simulink model "five_bar_discrete_model_v_1"  (R2018b)
settings: Solver=ode45  StartTime=0.0  StopTime=tmax-0.001  FixedStep=1e-4  MaxStep=1e-4  RelTol=1e-3
values from neighbouring files (symbols this model uses):
  dt = 10e-3    (= 0.01)    [model_parameters_v_1.m]    (also in test_dynamics.m = 0.2; test_kinematics.m = 0.1)
  dt_controller = 1e-3    (= 0.001)    [model_parameters_v_1.m]
  g = -9.80665    [idyn5.m]    (also in test_dynamics.m; test_model.m = 9.80665)
  Kd = (3*aj*wj-Fv) * eye(2)    [model_parameters_v_1.m]
  Kdi = [2 * zita *  wpos1; 2  * zita * wpos2]    [model_parameters_v_1.m]
  Ki = aj*wj^3 * eye(2)    [model_parameters_v_1.m]
  Kp = 3*aj*wj^2 * eye(2)    [model_parameters_v_1.m]
  Kpi = [ wpos1^2;  wpos2^2]    [model_parameters_v_1.m]
  lambda = 0.95    [model_parameters_v_1.m]
  p = [NaN; NaN]    [fkine5.m]    (also in test_model.m = zeros(n,2))
  q = [NaN; NaN; NaN; NaN; NaN]    [fkine5.m]    (also in ikine5.m = [q11;q12;q13;q21;q22])
  q0 = q(:,1)    [model_parameters_v_1.m]    (also in test_dynamics.m = q0(:,4); test_kinematics.m = q0(:,4))
  qd = [qda(1);qdu(1);qdu(2);qda(2);qdu(3)]    [ifirstkine5.m]
  qdd = [qdda(1);qddu(1);qddu(2);qdda(2);qddu(3)]    [isecondkine5.m]
  t0r = J * qda    [ffirstkine5.m]    (also in test_dynamics.m = [0;0]; test_kinematics.m = [1;1]; test_model.m = p)
  t0rd = (J * qdda+ at)    [fsecondkine5.m]    (also in test_dynamics.m = [0;0]; test_kinematics.m = [-1;1]; test_model.m = p)
undefined symbols (not defined in the file or in its folder): DiscIntNeverNeededParam, tmax, X, Y, Z
libraries: sm_lib x24, simulink x12, nesl_utility x9, commrandsrc3 x6, powerlib_meascontrol x2
(part 1 of 2)
settings Model: Creator=jere  LastModifiedBy=Jere
settings DebuggingCC: LibraryContextMissingDiagnostic=none
settings SFSimCC: SimUseLocalCustomCode=off
settings RTWCC: RTWUseLocalCustomCode=off

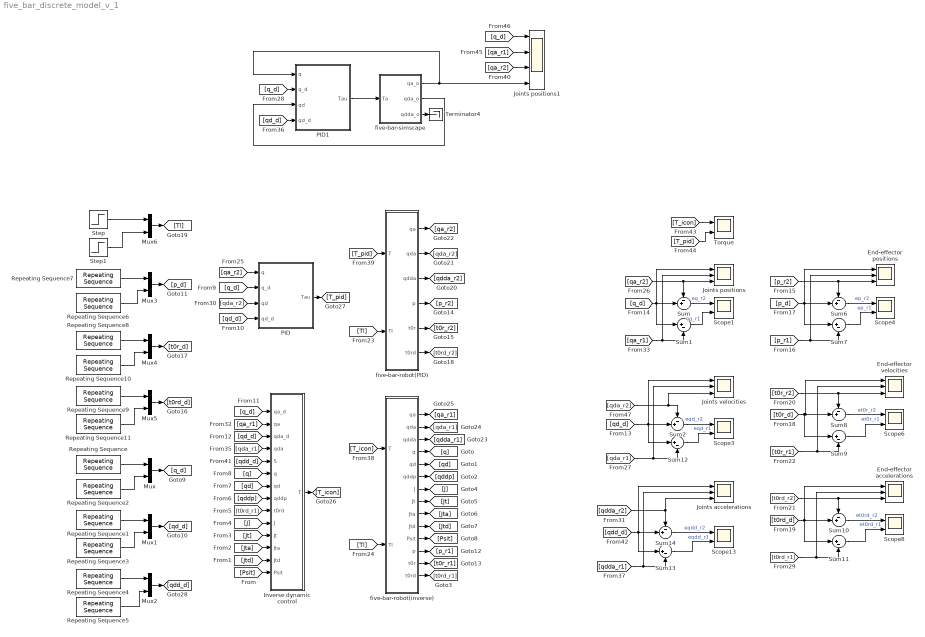
== system five_bar_discrete_model_v_1 ==
  End-effector accelerations : Scope  NumInputPorts=3
  End-effector positions : Scope  NumInputPorts=3
  End-effector velocities : Scope  NumInputPorts=3
  Inverse dynamic control : Subsystem
  Joints accelerations : Scope  NumInputPorts=3
  Joints positions : Scope  NumInputPorts=3
  Joints positions1 : Scope  NumInputPorts=4
  Joints velocities : Scope  NumInputPorts=3
  Mux{,1..6} (7 alike) : Mux  Inputs=2
  PID : Subsystem
  PID1 : Subsystem
  Repeating Sequence : simulink/Sources/Repeating Sequence  rep_seq_t=0:dt:tmax  rep_seq_y=q(1,:)
  Repeating Sequence1 : simulink/Sources/Repeating Sequence  rep_seq_t=0:dt:tmax  rep_seq_y=qd(1,:)
  Repeating Sequence10 : simulink/Sources/Repeating Sequence  rep_seq_t=0:dt:tmax  rep_seq_y=t0r(2,:)
  Repeating Sequence11 : simulink/Sources/Repeating Sequence  rep_seq_t=0:dt:tmax  rep_seq_y=t0rd(2,:)
  Repeating Sequence2 : simulink/Sources/Repeating Sequence  rep_seq_t=0:dt:tmax  rep_seq_y=q(4,:)
  Repeating Sequence3 : simulink/Sources/Repeating Sequence  rep_seq_t=0:dt:tmax  rep_seq_y=qd(4,:)
  Repeating Sequence4 : simulink/Sources/Repeating Sequence  rep_seq_t=0:dt:tmax  rep_seq_y=qdd(1,:)
  Repeating Sequence5 : simulink/Sources/Repeating Sequence  rep_seq_t=0:dt:tmax  rep_seq_y=qdd(4,:)
  Repeating Sequence6 : simulink/Sources/Repeating Sequence  rep_seq_t=0:dt:tmax  rep_seq_y=p(2,:)
  Repeating Sequence7 : simulink/Sources/Repeating Sequence  rep_seq_t=0:dt:tmax  rep_seq_y=p(1,:)
  Repeating Sequence8 : simulink/Sources/Repeating Sequence  rep_seq_t=0:dt:tmax  rep_seq_y=t0r(1,:)
  Repeating Sequence9 : simulink/Sources/Repeating Sequence  rep_seq_t=0:dt:tmax  rep_seq_y=t0rd(1,:)
  Scope{1,3..4,6,8,13} (6 alike) : Scope  NumInputPorts=2
  Step : Step  Time=tmax/2  SampleTime=0
  Step1 : Step  Time=tmax/2  SampleTime=0
  Sum{,2,6,8,10,14} (6 alike) : Sum  Inputs=-+|
  Sum{1,7,9,11..13} (6 alike) : Sum  Inputs=|+-
  Terminator4 : Terminator
  Torque : Scope  NumInputPorts=2
  five-bar-robot(PID) : Subsystem
  five-bar-robot(inverse) : Subsystem
  five-bar-simscape : Subsystem
  wires:
  Repeating Sequence/1 -> Mux/1
  Repeating Sequence2/1 -> Mux/2
  Repeating Sequence1/1 -> Mux1/1
  Repeating Sequence3/1 -> Mux1/2
  Repeating Sequence4/1 -> Mux2/1
  Repeating Sequence5/1 -> Mux2/2
  five-bar-robot(inverse)/4(q) -> [q]
  five-bar-robot(inverse)/5(qd) -> [qd]
  five-bar-robot(inverse)/6(qddp) -> [qddp]
  five-bar-robot(inverse)/14(t0rd) -> [t0rd_r1]
  five-bar-robot(inverse)/7(J) -> [J]
  five-bar-robot(inverse)/8(Jt) -> [Jt]
  five-bar-robot(inverse)/9(Jta) -> [Jta]
  five-bar-robot(inverse)/10(Jtd) -> [Jtd]
  five-bar-robot(inverse)/11(Psit) -> [Psit]
  [q] -> Inverse dynamic control/6(q)
  [qd] -> Inverse dynamic control/7(qd)
  [t0rd_r1] -> Inverse dynamic control/9(t0rd)
  [J] -> Inverse dynamic control/10(J)
  [Jt] -> Inverse dynamic control/11(Jt)
  [Jta] -> Inverse dynamic control/12(Jta)
  [Jtd] -> Inverse dynamic control/13(Jtd)
  [Psit] -> Inverse dynamic control/14(Psit)
  [qddp] -> Inverse dynamic control/8(qddp)
  five-bar-robot(PID)/1(qa) -> [qa_r2]
  Sum/1 -> Scope1/1  "eq_r2"
  Sum1/1 -> Scope1/2  "eq_r1"
  Mux/1 -> [q_d]
  [q_d] -> PID/2(q_d)
  Mux1/1 -> [qd_d]
  [qd_d] -> PID/4(qd_d)
  [qd_d] -> Inverse dynamic control/3(qda_d)
  [q_d] -> Inverse dynamic control/1(qa_d)
  Repeating Sequence6/1 -> Mux3/2
  Repeating Sequence7/1 -> Mux3/1
  Mux3/1 -> [p_d]
  five-bar-robot(inverse)/12(p) -> [p_r1]
  five-bar-robot(inverse)/13(t0r) -> [t0r_r1]
  five-bar-robot(PID)/4(p) -> [p_r2]
  five-bar-robot(PID)/5(t0r) -> [t0r_r2]
  Sum6/1 -> Scope4/1  "ep_r2"
  Sum7/1 -> Scope4/2  "ep_r1"
  [p_d] -> End-effector positions/1, Sum6/2, Sum7/1
  [p_r2] -> End-effector positions/3, Sum6/1
  [p_r1] -> End-effector positions/2, Sum7/2
  Repeating Sequence11/1 -> Mux5/2
  Repeating Sequence9/1 -> Mux5/1
  Repeating Sequence8/1 -> Mux4/1
  Mux5/1 -> [t0rd_d]
  Mux4/1 -> [t0r_d]
  Repeating Sequence10/1 -> Mux4/2
  five-bar-robot(PID)/6(t0rd) -> [t0rd_r2]
  [t0r_r1] -> End-effector velocities/2, Sum9/2
  Sum9/1 -> Scope6/2  "et0r_r1"
  [t0r_d] -> Sum9/1, End-effector velocities/1, Sum8/2
  [t0r_r2] -> End-effector velocities/3, Sum8/1
  Sum8/1 -> Scope6/1  "et0r_r2"
  [t0rd_r1] -> End-effector accelerations/2, Sum11/2
  Sum11/1 -> Scope8/2  "et0rd_r1"
  [t0rd_d] -> End-effector accelerations/1, Sum10/2, Sum11/1
  [t0rd_r2] -> End-effector accelerations/3, Sum10/1
  Sum10/1 -> Scope8/1  "et0rd_r2"
  five-bar-robot(PID)/3(qdda) -> [qdda_r2]
  [Tl] -> five-bar-robot(PID)/2(Tl)
  [Tl] -> five-bar-robot(inverse)/2(Tl)
  Step/1 -> Mux6/1
  Step1/1 -> Mux6/2
  Mux6/1 -> [Tl]
  [qa_r2] -> PID/1(q)
  [qa_r2] -> Sum/1, Joints positions/3
  five-bar-robot(PID)/2(qda) -> [qda_r2]
  [q_d] -> Sum/2, Sum1/1, Joints positions/1
  [qda_r2] -> PID/3(qd)
  five-bar-robot(inverse)/1(qa) -> [qa_r1]
  [qa_r1] -> Inverse dynamic control/2(qa)
  [qa_r1] -> Sum1/2, Joints positions/2
  [qda_r1] -> Joints velocities/2, Sum12/2
  five-bar-robot(inverse)/2(qda) -> [qda_r1]
  [qda_r1] -> Inverse dynamic control/4(qda)
  five-bar-robot(inverse)/3(qdda) -> [qdda_r1]
  Inverse dynamic control/1(T) -> [T_icon]
  [T_icon] -> five-bar-robot(inverse)/1(T)
  PID/1(Tau) -> [T_pid]
  [T_pid] -> five-bar-robot(PID)/1(T)
  Mux2/1 -> [qdd_d]
  [qdd_d] -> Inverse dynamic control/5(qdda_d)
  [T_icon] -> Torque/1
  [T_pid] -> Torque/2
  Sum2/1 -> Scope3/1  "eqd_r2"
  Sum12/1 -> Scope3/2  "eqd_r1"
  [qd_d] -> Sum2/2, Sum12/1, Joints velocities/1
  [qda_r2] -> Joints velocities/3, Sum2/1
  Sum13/1 -> Scope13/2  "eqdd_r1"
  [qdd_d] -> Sum13/1, Joints accelerations/1, Sum14/2
  [qdda_r1] -> Sum13/2, Joints accelerations/2
  Sum14/1 -> Scope13/1  "eqdd_r2"
  [qdda_r2] -> Sum14/1, Joints accelerations/3
  PID1/1(Tau) -> five-bar-simscape/1(Ta)
  five-bar-simscape/1(qa_o) -> Joints positions1/4, PID1/1(q)
  five-bar-simscape/2(qda_o) -> PID1/3(qd)
  [q_d] -> PID1/2(q_d)
  [qd_d] -> PID1/4(qd_d)
  [q_d] -> Joints positions1/1
  [qa_r1] -> Joints positions1/2
  [qa_r2] -> Joints positions1/3
  five-bar-simscape/3(qdda_o) -> Terminator4/1

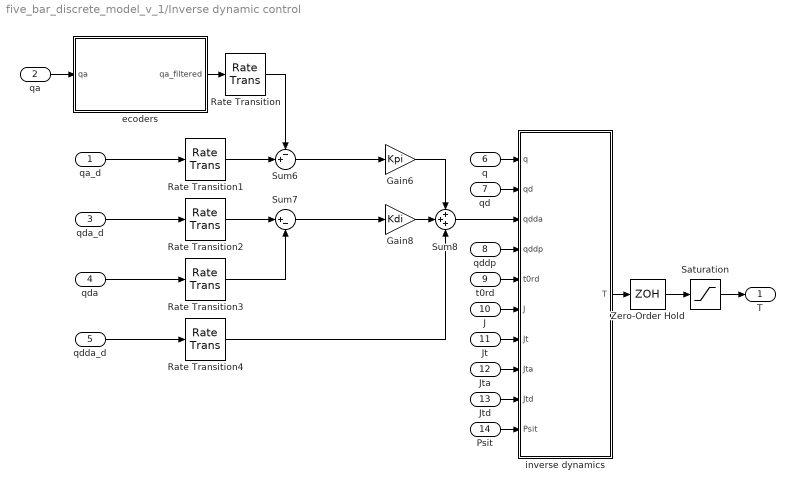
== system five_bar_discrete_model_v_1/Inverse dynamic control ==
  qa_d : Inport
  qa : Inport  Port=2
  qda_d : Inport  Port=3
  qda : Inport  Port=4
  qdda_d : Inport  Port=5
  q : Inport  Port=6
  qd : Inport  Port=7
  qddp : Inport  Port=8
  t0rd : Inport  Port=9
  J : Inport  Port=10
  Jt : Inport  Port=11
  Jta : Inport  Port=12
  Jtd : Inport  Port=13
  Psit : Inport  Port=14
  Gain6 : Gain  Gain=Kpi
  Gain8 : Gain  Gain=Kdi
  Rate Transition{,1..4} (5 alike) : RateTransition  InitialCondition=[q0(1);q0(4)]  OutPortSampleTime=dt_controller
  Saturation : Saturate  UpperLimit=3  LowerLimit=-3
  Sum6 : Sum  Inputs=-+|
  Sum7 : Sum  Inputs=|+-
  Sum8 : Sum  Inputs=+++
  Zero-Order Hold : ZeroOrderHold  SampleTime=dt_controller
  ecoders : Subsystem
  inverse dynamics : MATLAB Function  TreatAsAtomicUnit=on
  T : Outport
  wires:
  Psit/1 -> inverse dynamics/10(Psit)
  J/1 -> inverse dynamics/6(J)
  Sum7/1 -> Gain8/1
  Sum6/1 -> Gain6/1
  qa_d/1 -> Rate Transition1/1
  Jta/1 -> inverse dynamics/8(Jta)
  qd/1 -> inverse dynamics/2(qd)
  qddp/1 -> inverse dynamics/4(qddp)
  q/1 -> inverse dynamics/1(q)
  t0rd/1 -> inverse dynamics/5(t0rd)
  qdda_d/1 -> Rate Transition4/1
  inverse dynamics/1(T) -> Zero-Order Hold/1
  Jtd/1 -> inverse dynamics/9(Jtd)
  Jt/1 -> inverse dynamics/7(Jt)
  qda/1 -> Rate Transition3/1
  qda_d/1 -> Rate Transition2/1
  Gain8/1 -> Sum8/2
  Gain6/1 -> Sum8/1
  Saturation/1 -> T/1
  Sum8/1 -> inverse dynamics/3(qdda)
  Rate Transition/1 -> Sum6/1
  Rate Transition1/1 -> Sum6/2
  Rate Transition2/1 -> Sum7/1
  Rate Transition3/1 -> Sum7/2
  Rate Transition4/1 -> Sum8/3
  qa/1 -> ecoders/1(qa)
  ecoders/1(qa_filtered) -> Rate Transition/1
  Zero-Order Hold/1 -> Saturation/1

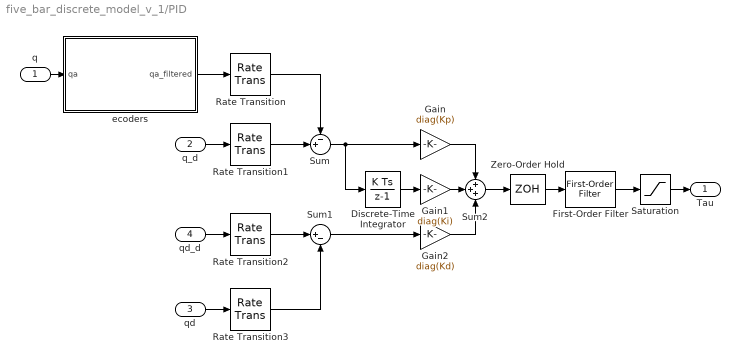
== system five_bar_discrete_model_v_1/PID ==
  q : Inport
  q_d : Inport  Port=2
  qd : Inport  Port=3
  qd_d : Inport  Port=4
  Discrete-Time Integrator : DiscreteIntegrator  InitialCondition=[0;0]  SampleTime=dt_controller  ICPrevOutput=DiscIntNeverNeededParam  ICPrevScaledInput=DiscIntNeverNeededParam
  First-Order Filter : powerlib_meascontrol/Filters/First-Order Filter  FilterType=Lowpass  Tc=0.006  Ts=dt_controller  Initialize=off  Vac_Init=[0, 0, 60]  Vdc_Init=0  PlotResponse=off  FreqRange="[0,  200,  1]"
      settings: SourceProductName=Simscape Electrical
  Gain : Gain  Gain=diag(Kp)
  Gain1 : Gain  Gain=diag(Ki)
  Gain2 : Gain  Gain=diag(Kd)
  Rate Transition{,1..3} (4 alike) : RateTransition  InitialCondition=[q0(1);q0(4)]  OutPortSampleTime=dt_controller
  Saturation : Saturate  UpperLimit=2  LowerLimit=-2
  Sum : Sum  Inputs=-+|
  Sum1 : Sum  Inputs=|+-
  Sum2 : Sum  Inputs=+++
  Zero-Order Hold : ZeroOrderHold  SampleTime=dt_controller
  ecoders : Subsystem
  Tau : Outport
  wires:
  Gain/1 -> Sum2/1
  Sum/1 -> Discrete-Time Integrator/1, Gain/1
  Gain1/1 -> Sum2/2
  q_d/1 -> Rate Transition1/1
  qd_d/1 -> Rate Transition2/1
  Sum2/1 -> Zero-Order Hold/1
  Sum1/1 -> Gain2/1
  qd/1 -> Rate Transition3/1
  Gain2/1 -> Sum2/3
  First-Order Filter/1 -> Saturation/1
  Saturation/1 -> Tau/1
  Rate Transition1/1 -> Sum/2
  Rate Transition2/1 -> Sum1/1
  Rate Transition3/1 -> Sum1/2
  Zero-Order Hold/1 -> First-Order Filter/1
  Discrete-Time Integrator/1 -> Gain1/1
  Rate Transition/1 -> Sum/1
  q/1 -> ecoders/1(qa)
  ecoders/1(qa_filtered) -> Rate Transition/1

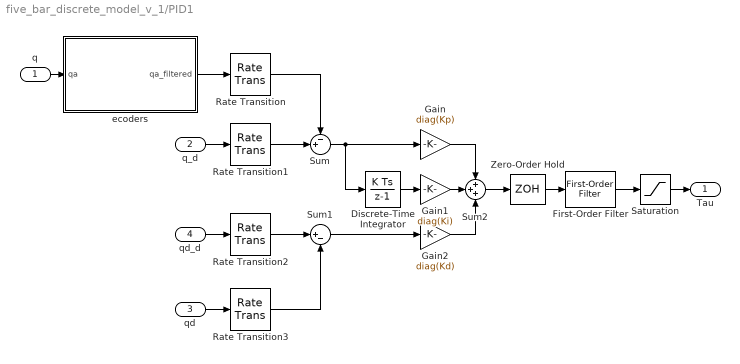
== system five_bar_discrete_model_v_1/PID1 ==
  q : Inport
  q_d : Inport  Port=2
  qd : Inport  Port=3
  qd_d : Inport  Port=4
  Discrete-Time Integrator : DiscreteIntegrator  InitialCondition=[0;0]  SampleTime=dt_controller  ICPrevOutput=DiscIntNeverNeededParam  ICPrevScaledInput=DiscIntNeverNeededParam
  First-Order Filter : powerlib_meascontrol/Filters/First-Order Filter  FilterType=Lowpass  Tc=0.006  Ts=dt_controller  Initialize=off  Vac_Init=[0, 0, 60]  Vdc_Init=0  PlotResponse=off  FreqRange="[0,  200,  1]"
      settings: SourceProductName=Simscape Electrical
  Gain : Gain  Gain=diag(Kp)
  Gain1 : Gain  Gain=diag(Ki)
  Gain2 : Gain  Gain=diag(Kd)
  Rate Transition{,1..3} (4 alike) : RateTransition  InitialCondition=[q0(1);q0(4)]  OutPortSampleTime=dt_controller
  Saturation : Saturate  UpperLimit=2  LowerLimit=-2
  Sum : Sum  Inputs=-+|
  Sum1 : Sum  Inputs=|+-
  Sum2 : Sum  Inputs=+++
  Zero-Order Hold : ZeroOrderHold  SampleTime=dt_controller
  ecoders : Subsystem
  Tau : Outport
  wires:
  Gain/1 -> Sum2/1
  Sum/1 -> Discrete-Time Integrator/1, Gain/1
  Gain1/1 -> Sum2/2
  q_d/1 -> Rate Transition1/1
  qd_d/1 -> Rate Transition2/1
  Sum2/1 -> Zero-Order Hold/1
  Sum1/1 -> Gain2/1
  qd/1 -> Rate Transition3/1
  Gain2/1 -> Sum2/3
  First-Order Filter/1 -> Saturation/1
  Saturation/1 -> Tau/1
  Rate Transition1/1 -> Sum/2
  Rate Transition2/1 -> Sum1/1
  Rate Transition3/1 -> Sum1/2
  Zero-Order Hold/1 -> First-Order Filter/1
  Discrete-Time Integrator/1 -> Gain1/1
  Rate Transition/1 -> Sum/1
  q/1 -> ecoders/1(qa)
  ecoders/1(qa_filtered) -> Rate Transition/1

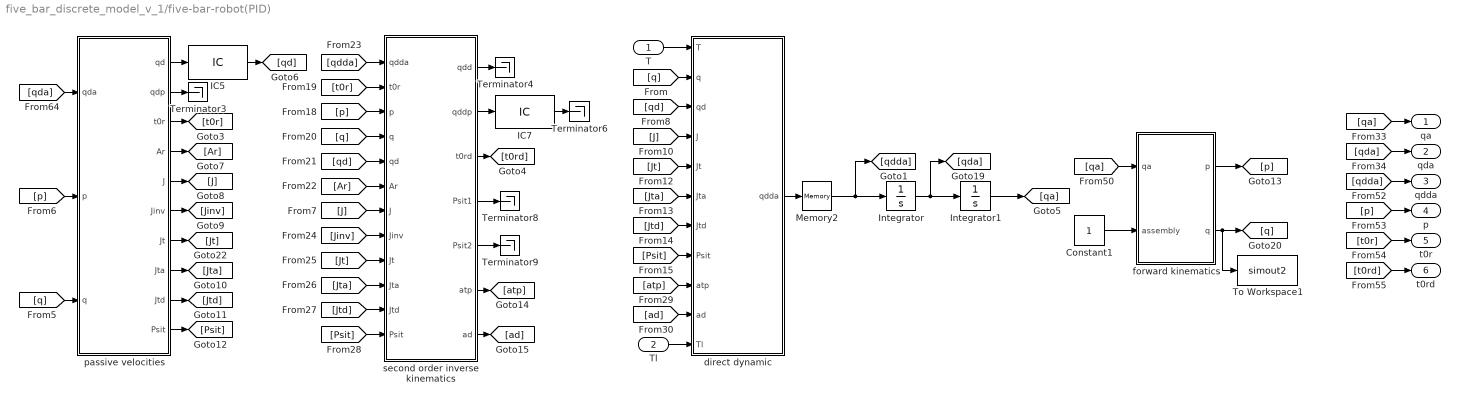
== system five_bar_discrete_model_v_1/five-bar-robot(PID) ==
  T : Inport
  Tl : Inport  Port=2
  Constant1 : Constant
  IC5 : InitialCondition  Value=zeros(5,1)
  IC7 : InitialCondition  Value=zeros(3,1)
  Integrator : Integrator  InitialCondition=[0;0]
  Integrator1 : Integrator  InitialCondition=[q0(1);q0(4)]
  Memory2 : Memory  InitialCondition=[0;0]
  Terminator{3..4,6,8..9} (5 alike) : Terminator
  To Workspace1 : ToWorkspace  VariableName=simout2  SaveFormat=Timeseries  SampleTime=-1
  direct dynamic : MATLAB Function  TreatAsAtomicUnit=on
  forward kinematics : MATLAB Function  TreatAsAtomicUnit=on
  passive velocities : MATLAB Function  TreatAsAtomicUnit=on
  second order inverse kinematics : MATLAB Function  TreatAsAtomicUnit=on
  qa : Outport
  qda : Outport  Port=2
  qdda : Outport  Port=3
  p : Outport  Port=4
  t0r : Outport  Port=5
  t0rd : Outport  Port=6
  wires:
  [qdda] -> qdda/1
  [qa] -> forward kinematics/1(qa)
  forward kinematics/1(p) -> [p]
  forward kinematics/2(q) -> To Workspace1/1, [q]
  Constant1/1 -> forward kinematics/2(assembly)
  [qda] -> qda/1
  [p] -> p/1
  [t0r] -> t0r/1
  [t0rd] -> t0rd/1
  [Jt] -> second order inverse kinematics/9(Jt)
  [Jtd] -> second order inverse kinematics/11(Jtd)
  [p] -> passive velocities/2(p)
  [qd] -> second order inverse kinematics/5(qd)
  Integrator1/1 -> [qa]
  second order inverse kinematics/5(Psit2) -> Terminator9/1
  passive velocities/3(t0r) -> [t0r]
  [Jta] -> second order inverse kinematics/10(Jta)
  [atp] -> direct dynamic/9(atp)
  T/1 -> direct dynamic/1(T)
  second order inverse kinematics/7(ad) -> [ad]
  passive velocities/1(qd) -> IC5/1
  second order inverse kinematics/4(Psit1) -> Terminator8/1
  Integrator/1 -> [qda], Integrator1/1
  passive velocities/6(Jinv) -> [Jinv]
  [J] -> second order inverse kinematics/7(J)
  passive velocities/8(Jta) -> [Jta]
  [Ar] -> second order inverse kinematics/6(Ar)
  second order inverse kinematics/6(atp) -> [atp]
  passive velocities/4(Ar) -> [Ar]
  [Jta] -> direct dynamic/6(Jta)
  [qdda] -> second order inverse kinematics/1(qdda)
  [qda] -> passive velocities/1(qda)
  [q] -> second order inverse kinematics/4(q)
  [p] -> second order inverse kinematics/3(p)
  Memory2/1 -> Integrator/1, [qdda]
  IC7/1 -> Terminator6/1
  [t0r] -> second order inverse kinematics/2(t0r)
  [q] -> direct dynamic/2(q)
  second order inverse kinematics/3(t0rd) -> [t0rd]
  passive velocities/7(Jt) -> [Jt]
  [q] -> passive velocities/3(q)
  [Jt] -> direct dynamic/5(Jt)
  Tl/1 -> direct dynamic/11(Tl)
  [ad] -> direct dynamic/10(ad)
  [qd] -> direct dynamic/3(qd)
  passive velocities/10(Psit) -> [Psit]
  [Jtd] -> direct dynamic/7(Jtd)
  passive velocities/2(qdp) -> Terminator3/1
  [Psit] -> second order inverse kinematics/12(Psit)
  direct dynamic/1(qdda) -> Memory2/1
  second order inverse kinematics/2(qddp) -> IC7/1
  [Jinv] -> second order inverse kinematics/8(Jinv)
  [Psit] -> direct dynamic/8(Psit)
  IC5/1 -> [qd]
  [J] -> direct dynamic/4(J)
  second order inverse kinematics/1(qdd) -> Terminator4/1
  passive velocities/5(J) -> [J]
  passive velocities/9(Jtd) -> [Jtd]
  [qa] -> qa/1

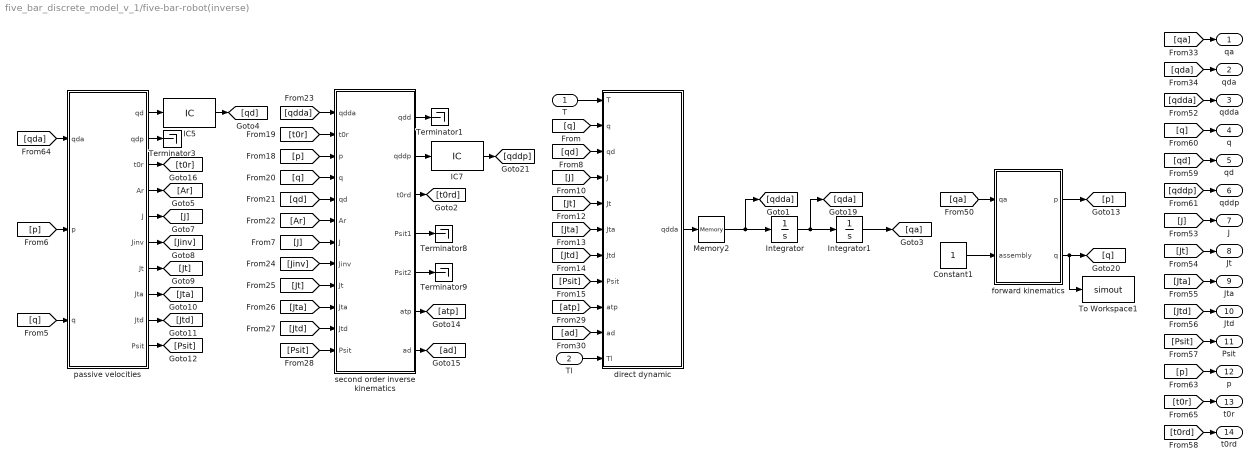
== system five_bar_discrete_model_v_1/five-bar-robot(inverse) ==
  T : Inport
  Tl : Inport  Port=2
  Constant1 : Constant
  IC5 : InitialCondition  Value=zeros(5,1)
  IC7 : InitialCondition  Value=zeros(3,1)
  Integrator : Integrator  InitialCondition=[0;0]
  Integrator1 : Integrator  InitialCondition=[q0(1);q0(4)]
  Memory2 : Memory  InitialCondition=[0;0]
  Terminator{1,3,8..9} (4 alike) : Terminator
  To Workspace1 : ToWorkspace  VariableName=simout  SaveFormat=Timeseries  SampleTime=-1
  direct dynamic : MATLAB Function  TreatAsAtomicUnit=on
  forward kinematics : MATLAB Function  TreatAsAtomicUnit=on
  passive velocities : MATLAB Function  TreatAsAtomicUnit=on
  second order inverse kinematics : MATLAB Function  TreatAsAtomicUnit=on
  qa : Outport
  qda : Outport  Port=2
  qdda : Outport  Port=3
  q : Outport  Port=4
  qd : Outport  Port=5
  qddp : Outport  Port=6
  J : Outport  Port=7
  Jt : Outport  Port=8
  Jta : Outport  Port=9
  Jtd : Outport  Port=10
  Psit : Outport  Port=11
  p : Outport  Port=12
  t0r : Outport  Port=13
  t0rd : Outport  Port=14
  wires:
  [p] -> second order inverse kinematics/3(p)
  second order inverse kinematics/6(atp) -> [atp]
  [ad] -> direct dynamic/10(ad)
  [Psit] -> second order inverse kinematics/12(Psit)
  [q] -> second order inverse kinematics/4(q)
  passive velocities/7(Jt) -> [Jt]
  [qd] -> direct dynamic/3(qd)
  [Psit] -> direct dynamic/8(Psit)
  [Jinv] -> second order inverse kinematics/8(Jinv)
  passive velocities/10(Psit) -> [Psit]
  Integrator1/1 -> [qa]
  passive velocities/4(Ar) -> [Ar]
  second order inverse kinematics/5(Psit2) -> Terminator9/1
  second order inverse kinematics/7(ad) -> [ad]
  [qdda] -> qdda/1
  [qd] -> second order inverse kinematics/5(qd)
  [Jta] -> direct dynamic/6(Jta)
  [q] -> direct dynamic/2(q)
  passive velocities/5(J) -> [J]
  passive velocities/6(Jinv) -> [Jinv]
  [qa] -> forward kinematics/1(qa)
  second order inverse kinematics/4(Psit1) -> Terminator8/1
  forward kinematics/1(p) -> [p]
  forward kinematics/2(q) -> To Workspace1/1, [q]
  passive velocities/9(Jtd) -> [Jtd]
  [Jta] -> second order inverse kinematics/10(Jta)
  [Jt] -> second order inverse kinematics/9(Jt)
  [t0r] -> second order inverse kinematics/2(t0r)
  Constant1/1 -> forward kinematics/2(assembly)
  [J] -> direct dynamic/4(J)
  [qa] -> qa/1
  [Jt] -> direct dynamic/5(Jt)
  [Ar] -> second order inverse kinematics/6(Ar)
  [Jtd] -> direct dynamic/7(Jtd)
  Integrator/1 -> [qda], Integrator1/1
  passive velocities/1(qd) -> IC5/1
  [q] -> passive velocities/3(q)
  passive velocities/8(Jta) -> [Jta]
  [p] -> passive velocities/2(p)
  [qda] -> qda/1
  passive velocities/2(qdp) -> Terminator3/1
  IC5/1 -> [qd]
  [Jtd] -> second order inverse kinematics/11(Jtd)
  T/1 -> direct dynamic/1(T)
  [atp] -> direct dynamic/9(atp)
  [q] -> q/1
  [qd] -> qd/1
  [qddp] -> qddp/1
  [t0rd] -> t0rd/1
  [J] -> J/1
  [Jt] -> Jt/1
  [Jta] -> Jta/1
  [Jtd] -> Jtd/1
  [Psit] -> Psit/1
  direct dynamic/1(qdda) -> Memory2/1
  [p] -> p/1
  [t0r] -> t0r/1
  Tl/1 -> direct dynamic/11(Tl)
  [qda] -> passive velocities/1(qda)
  [qdda] -> second order inverse kinematics/1(qdda)
  passive velocities/3(t0r) -> [t0r]
  [J] -> second order inverse kinematics/7(J)
  second order inverse kinematics/3(t0rd) -> [t0rd]
  second order inverse kinematics/2(qddp) -> IC7/1
  IC7/1 -> [qddp]
  Memory2/1 -> Integrator/1, [qdda]
  second order inverse kinematics/1(qdd) -> Terminator1/1

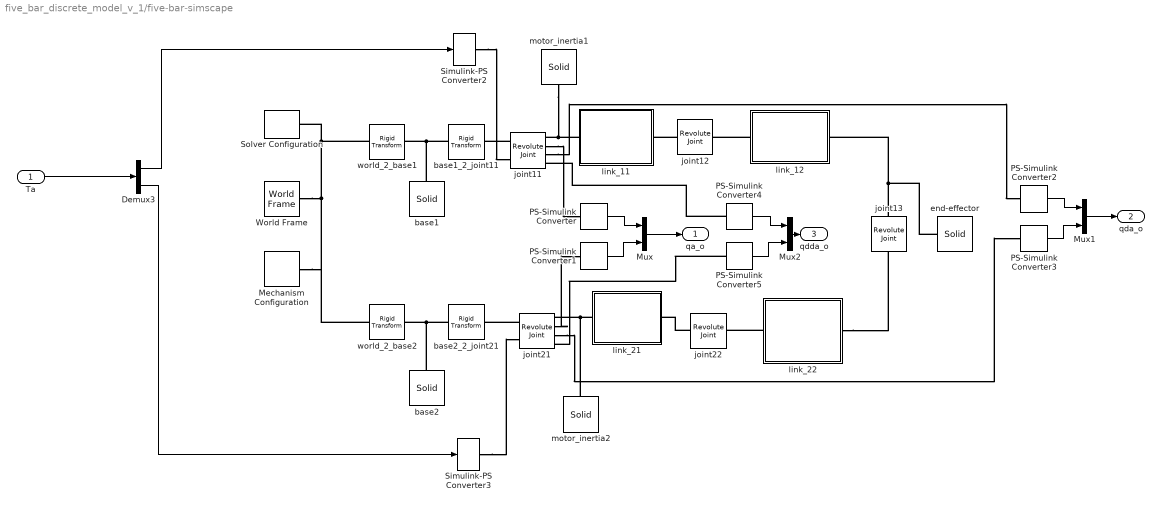
== system five_bar_discrete_model_v_1/five-bar-simscape ==
  Ta : Inport
  Demux3 : Demux  Outputs=2
  Mechanism Configuration : sm_lib/Utilities/Mechanism Configuration  UniformGravity=Constant  GravityVector=[0 0 0]  GravityUnits=m/s^2  LinearizationDelta=0.001
  Mux : Mux  Inputs=2
  Mux1 : Mux  Inputs=2
  Mux2 : Mux  Inputs=2
  PS-Simulink Converter : nesl_utility/PS-Simulink Converter  PhysicalDomain=network_engine_domain  SubClassName=ps_output  LeftPortType=input  RightPortType=output  PseudoPeriodic=off  Frequencies=[]  Unit=rad  AffineConversion=off
  PS-Simulink Converter1 : nesl_utility/PS-Simulink Converter  PhysicalDomain=network_engine_domain  SubClassName=ps_output  LeftPortType=input  RightPortType=output  PseudoPeriodic=off  Frequencies=[]  Unit=rad  AffineConversion=off
  PS-Simulink Converter{2..5} (4 alike) : nesl_utility/PS-Simulink Converter  PhysicalDomain=network_engine_domain  SubClassName=ps_output  LeftPortType=input  RightPortType=output  PseudoPeriodic=off  Frequencies=[]  Unit=1  AffineConversion=off
  Simulink-PS Converter2 : nesl_utility/Simulink-PS Converter  PhysicalDomain=network_engine_domain  SubClassName=ps_input  LeftPortType=input  RightPortType=output  PseudoPeriodic=off  Frequencies=[]  NoiseDistribution=none  NoiseParameters=[]  Unit=N*m  AffineConversion=off  FilteringAndDerivatives=provide  SimscapeFilterOrder=1  InputFilterTimeConstant=0.001  UdotUserProvided=0
  Simulink-PS Converter3 : nesl_utility/Simulink-PS Converter  PhysicalDomain=network_engine_domain  SubClassName=ps_input  LeftPortType=input  RightPortType=output  PseudoPeriodic=off  Frequencies=[]  NoiseDistribution=none  NoiseParameters=[]  Unit=N*m  AffineConversion=off  FilteringAndDerivatives=provide  SimscapeFilterOrder=1  InputFilterTimeConstant=0.001  UdotUserProvided=0
  Solver Configuration : nesl_utility/Solver Configuration  PhysicalDomain=network_engine_domain  SubClassName=solver  LeftPortType=input  RightPortType=generic  Tones=[]  Harmonics=[]  SimulateNoise=off  Profile=off  UseLocalSampling=off  EnableSwitchedLinearOptims=on  FrequencyDomain=off  UseCCode=off  RelTol=0.001  AbsTol=1e-06  MinStep=1e-09  ToWorkspace=off  RevertToSquareIcSolve=off  NumHomotopyIterations=100  PhasorMode=off  PhasorModeNumHarmonics=1  DoDC=off  ResidualTolerance=1e-09  UseLocalSolver=off  LocalSolverChoice=NE_BACKWARD_EULER_ADVANCER  LocalSolverSampleTime=0.001  DoFixedCost=off  MaxNonlinIter=3  MaxModeIter=2  LinearAlgebra=Sparse  EquationFormulation=NE_TIME_EF  DelaysMemoryBudget=1024  AutomaticFiltering=on  FilteringTimeConstant=0.001  PartitionStorageMethod=AS_NEEDED  PartitionMemoryBudget=1024
  World Frame : sm_lib/Frames and Transforms/World Frame
  base1 : sm_lib/Body Elements/Solid  InertiaType=PointMass  Mass=1.72  MassUnits=kg  CenterOfMass=[0 0 0]  CenterOfMassUnits=m  MomentsOfInertia=[1 1 1]  MomentsOfInertiaUnits=kg*m^2  ProductsOfInertia=[0 0 0]  ProductsOfInertiaUnits=kg*m^2  BasedOnType=Density  Density=1000  DensityUnits=kg/m^3  DoExposeReferenceFrame=on  SerializedFrames=<Frames/>  GraphicType=FromGeometry  MarkerShape=Sphere  MarkerSize=10  GraphicVisPropType=SimpleVisualProperties  GraphicDiffuseColor=[1.0 1.0 0.0]  GraphicSpecularColor=[0.5 0.5 0.5 1.0]  GraphicAmbientColor=[0.15 0.15 0.15 1.0]  GraphicEmissiveColor=[0.0 0.0 0.0 1.0]  GraphicShininess=75  GraphicOpacity=1.0  GeometryShape=FromFile  RectangleSize=[1 1]  RectangleSizeUnits=m  BrickDimensions=[1 1 1]  BrickDimensionUnits=m  CylinderRadius=1  CylinderRadiusUnits=m  CylinderLength=1  CylinderLengthUnits=m  SphereRadius=1  SphereRadiusUnits=m  EllipsoidRadii=[1 1 1]  EllipsoidRadiiUnits=m  ExtrusionCrossSection=[1 1; -1 1; -1 -1; 1 -1]  ExtrusionCrossSectionUnits=m  ExtrusionLength=1  ExtrusionLengthUnits=m  PolygonNumSides=3  PolygonOuterRadius=1  PolygonOuterRadiusUnits=m  ExtGeomFileType=STL  ExtGeomFileName=/home/jere/Documentos/simulacionPF/5-bar-model/meshes/nema23_75mm_8mm.stl  ExtGeomFileUnits=mm  RevolutionCrossSection=[1 1; 1 -1; 2 -1; 2 1]  RevolutionCrossSectionUnits=m  RevolutionExtent=Full  RevolutionAngle=180  RevolutionAngleUnits=deg
  base1_2_joint11 : sm_lib/Frames and Transforms/Rigid Transform  TranslationMethod=Cartesian  TranslationStandardOffset=0  TranslationLengthUnit=mm  TranslationStandardAxis=+Z  TranslationCartesianOffset=[0 0 2]  TranslationROffset=0  TranslationROffsetUnits=m  TranslationZOffset=0  TranslationZOffsetUnits=m  TranslationThetaOffset=0  TranslationThetaOffsetUnits=deg  RotationMethod=None  RotationAngleUnits=deg  RotationStandardAxis=+Z  RotationAngle=0.0  RotationArbitraryAxis=[0 0 1]  FollAlignAxisA=+X  BaseAlignAxisA=+Y  FollAlignAxisB=+Y  BaseAlignAxisB=+Z  RotationSequenceAxes=FollowerAxes  RotationSequence=XYX  RotationSequenceAngles=[0 0 0]  RotationSequenceAnglesUnits=deg  RotationMatrix=[1 0 0; 0 1 0; 0 0 1]
  base2 : sm_lib/Body Elements/Solid  InertiaType=PointMass  Mass=1.72  MassUnits=kg  CenterOfMass=[0 0 0]  CenterOfMassUnits=m  MomentsOfInertia=[1 1 1]  MomentsOfInertiaUnits=kg*m^2  ProductsOfInertia=[0 0 0]  ProductsOfInertiaUnits=kg*m^2  BasedOnType=Density  Density=1000  DensityUnits=kg/m^3  DoExposeReferenceFrame=on  SerializedFrames=<Frames/>  GraphicType=FromGeometry  MarkerShape=Sphere  MarkerSize=10  GraphicVisPropType=SimpleVisualProperties  GraphicDiffuseColor=[1.0 1.0 0.0]  GraphicSpecularColor=[0.5 0.5 0.5 1.0]  GraphicAmbientColor=[0.15 0.15 0.15 1.0]  GraphicEmissiveColor=[0.0 0.0 0.0 1.0]  GraphicShininess=75  GraphicOpacity=1.0  GeometryShape=FromFile  RectangleSize=[1 1]  RectangleSizeUnits=m  BrickDimensions=[1 1 1]  BrickDimensionUnits=m  CylinderRadius=1  CylinderRadiusUnits=m  CylinderLength=1  CylinderLengthUnits=m  SphereRadius=1  SphereRadiusUnits=m  EllipsoidRadii=[1 1 1]  EllipsoidRadiiUnits=m  ExtrusionCrossSection=[1 1; -1 1; -1 -1; 1 -1]  ExtrusionCrossSectionUnits=m  ExtrusionLength=1  ExtrusionLengthUnits=m  PolygonNumSides=3  PolygonOuterRadius=1  PolygonOuterRadiusUnits=m  ExtGeomFileType=STL  ExtGeomFileName=/home/jere/Documentos/simulacionPF/5-bar-model/meshes/nema23_75mm_8mm.stl  ExtGeomFileUnits=mm  RevolutionCrossSection=[1 1; 1 -1; 2 -1; 2 1]  RevolutionCrossSectionUnits=m  RevolutionExtent=Full  RevolutionAngle=180  RevolutionAngleUnits=deg
  base2_2_joint21 : sm_lib/Frames and Transforms/Rigid Transform  TranslationMethod=Cartesian  TranslationStandardOffset=0  TranslationLengthUnit=mm  TranslationStandardAxis=+Z  TranslationCartesianOffset=[0 0 2]  TranslationROffset=0  TranslationROffsetUnits=m  TranslationZOffset=0  TranslationZOffsetUnits=m  TranslationThetaOffset=0  TranslationThetaOffsetUnits=deg  RotationMethod=None  RotationAngleUnits=deg  RotationStandardAxis=+Z  RotationAngle=0.0  RotationArbitraryAxis=[0 0 1]  FollAlignAxisA=+X  BaseAlignAxisA=+Y  FollAlignAxisB=+Y  BaseAlignAxisB=+Z  RotationSequenceAxes=FollowerAxes  RotationSequence=XYX  RotationSequenceAngles=[0 0 0]  RotationSequenceAnglesUnits=deg  RotationMatrix=[1 0 0; 0 1 0; 0 0 1]
  end-effector : sm_lib/Body Elements/Solid  InertiaType=PointMass  Mass=0.272  MassUnits=kg  CenterOfMass=[0 0 0]  CenterOfMassUnits=m  MomentsOfInertia=[1 1 1]  MomentsOfInertiaUnits=kg*m^2  ProductsOfInertia=[0 0 0]  ProductsOfInertiaUnits=kg*m^2  BasedOnType=Density  Density=1000  DensityUnits=kg/m^3  DoExposeReferenceFrame=on  SerializedFrames=<Frames/>  GraphicType=FromGeometry  MarkerShape=Sphere  MarkerSize=10  GraphicVisPropType=SimpleVisualProperties  GraphicDiffuseColor=[1.0 1.0 0.0]  GraphicSpecularColor=[0.5 0.5 0.5 1.0]  GraphicAmbientColor=[0.15 0.15 0.15 1.0]  GraphicEmissiveColor=[0.0 0.0 0.0 1.0]  GraphicShininess=75  GraphicOpacity=1.0  GeometryShape=Sphere  RectangleSize=[1 1]  RectangleSizeUnits=m  BrickDimensions=[1 1 1]  BrickDimensionUnits=m  CylinderRadius=1  CylinderRadiusUnits=m  CylinderLength=1  CylinderLengthUnits=m  SphereRadius=1  SphereRadiusUnits=mm  EllipsoidRadii=[1 1 1]  EllipsoidRadiiUnits=m  ExtrusionCrossSection=[1 1; -1 1; -1 -1; 1 -1]  ExtrusionCrossSectionUnits=m  ExtrusionLength=1  ExtrusionLengthUnits=m  PolygonNumSides=3  PolygonOuterRadius=1  PolygonOuterRadiusUnits=m  ExtGeomFileType=STL  ExtGeomFileName=D:\PartsMechanism\propiedades\nema23_75mm_8mm.stl  ExtGeomFileUnits=mm  RevolutionCrossSection=[1 1; 1 -1; 2 -1; 2 1]  RevolutionCrossSectionUnits=m  RevolutionExtent=Full  RevolutionAngle=180  RevolutionAngleUnits=deg
  joint11 : sm_lib/Joints/Revolute Joint  SenseConstraintForce=off  SenseConstraintForceX=off  SenseConstraintForceY=off  SenseConstraintForceZ=off  SenseConstraintTorque=off  SenseConstraintTorqueX=off  SenseConstraintTorqueY=off  SenseConstraintTorqueZ=off  SenseTotalForce=off  SenseTotalForceX=off  SenseTotalForceY=off  SenseTotalForceZ=off  SenseTotalTorque=off  SenseTotalTorqueX=off  SenseTotalTorqueY=off  SenseTotalTorqueZ=off  CompositeWrenchDir=FollowerOnBase  CompositeWrenchFrame=BaseFrame  EquilibriumPosition=0  EquilibriumPositionUnits=rad  SpringStiffness=0  SpringStiffnessUnits=N*m/deg  DampingCoefficient=1.5e-1  DampingCoefficientUnits=N*m/(rad/s)  TorqueActuationMode=InputTorque  MotionActuationMode=ComputedMotion  SensePosition=on  SenseVelocity=on  SenseAcceleration=on  SenseTorqueForce=off  PositionTargetSpecify=on  PositionTargetPriority=High  PositionTargetValue=q(1,1)  PositionTargetValueUnits=rad  VelocityTargetSpecify=off  VelocityTargetPriority=High  VelocityTargetValue=1  VelocityTargetValueUnits=rad/s
  joint12 : sm_lib/Joints/Revolute Joint  SenseConstraintForce=off  SenseConstraintForceX=off  SenseConstraintForceY=off  SenseConstraintForceZ=off  SenseConstraintTorque=off  SenseConstraintTorqueX=off  SenseConstraintTorqueY=off  SenseConstraintTorqueZ=off  SenseTotalForce=off  SenseTotalForceX=off  SenseTotalForceY=off  SenseTotalForceZ=off  SenseTotalTorque=off  SenseTotalTorqueX=off  SenseTotalTorqueY=off  SenseTotalTorqueZ=off  CompositeWrenchDir=FollowerOnBase  CompositeWrenchFrame=BaseFrame  EquilibriumPosition=0  EquilibriumPositionUnits=rad  SpringStiffness=0  SpringStiffnessUnits=N*m/deg  DampingCoefficient=0  DampingCoefficientUnits=N*m/(rad/s)  TorqueActuationMode=NoTorque  MotionActuationMode=ComputedMotion  SensePosition=off  SenseVelocity=off  SenseAcceleration=off  SenseTorqueForce=off  PositionTargetSpecify=off  PositionTargetPriority=High  PositionTargetValue=q(2,1)  PositionTargetValueUnits=rad  VelocityTargetSpecify=off  VelocityTargetPriority=High  VelocityTargetValue=100  VelocityTargetValueUnits=rad/s
  joint13 : sm_lib/Joints/Revolute Joint  SenseConstraintForce=off  SenseConstraintForceX=off  SenseConstraintForceY=off  SenseConstraintForceZ=off  SenseConstraintTorque=off  SenseConstraintTorqueX=off  SenseConstraintTorqueY=off  SenseConstraintTorqueZ=off  SenseTotalForce=off  SenseTotalForceX=off  SenseTotalForceY=off  SenseTotalForceZ=off  SenseTotalTorque=off  SenseTotalTorqueX=off  SenseTotalTorqueY=off  SenseTotalTorqueZ=off  CompositeWrenchDir=FollowerOnBase  CompositeWrenchFrame=BaseFrame  EquilibriumPosition=0  EquilibriumPositionUnits=rad  SpringStiffness=0  SpringStiffnessUnits=N*m/deg  DampingCoefficient=0  DampingCoefficientUnits=N*m/(rad/s)  TorqueActuationMode=NoTorque  MotionActuationMode=ComputedMotion  SensePosition=off  SenseVelocity=off  SenseAcceleration=off  SenseTorqueForce=off  PositionTargetSpecify=off  PositionTargetPriority=High  PositionTargetValue=270  PositionTargetValueUnits=rad  VelocityTargetSpecify=off  VelocityTargetPriority=High  VelocityTargetValue=100  VelocityTargetValueUnits=rad/s
  joint21 : sm_lib/Joints/Revolute Joint  SenseConstraintForce=off  SenseConstraintForceX=off  SenseConstraintForceY=off  SenseConstraintForceZ=off  SenseConstraintTorque=off  SenseConstraintTorqueX=off  SenseConstraintTorqueY=off  SenseConstraintTorqueZ=off  SenseTotalForce=off  SenseTotalForceX=off  SenseTotalForceY=off  SenseTotalForceZ=off  SenseTotalTorque=off  SenseTotalTorqueX=off  SenseTotalTorqueY=off  SenseTotalTorqueZ=off  CompositeWrenchDir=FollowerOnBase  CompositeWrenchFrame=BaseFrame  EquilibriumPosition=0  EquilibriumPositionUnits=rad  SpringStiffness=0  SpringStiffnessUnits=N*m/deg  DampingCoefficient=1.5e-1  DampingCoefficientUnits=N*m/(rad/s)  TorqueActuationMode=InputTorque  MotionActuationMode=ComputedMotion  SensePosition=on  SenseVelocity=on  SenseAcceleration=on  SenseTorqueForce=off  PositionTargetSpecify=on  PositionTargetPriority=High  PositionTargetValue=q(4,1)  PositionTargetValueUnits=rad  VelocityTargetSpecify=off  VelocityTargetPriority=High  VelocityTargetValue=100  VelocityTargetValueUnits=rad/s
  joint22 : sm_lib/Joints/Revolute Joint  SenseConstraintForce=off  SenseConstraintForceX=off  SenseConstraintForceY=off  SenseConstraintForceZ=off  SenseConstraintTorque=off  SenseConstraintTorqueX=off  SenseConstraintTorqueY=off  SenseConstraintTorqueZ=off  SenseTotalForce=off  SenseTotalForceX=off  SenseTotalForceY=off  SenseTotalForceZ=off  SenseTotalTorque=off  SenseTotalTorqueX=off  SenseTotalTorqueY=off  SenseTotalTorqueZ=off  CompositeWrenchDir=FollowerOnBase  CompositeWrenchFrame=BaseFrame  EquilibriumPosition=0  EquilibriumPositionUnits=rad  SpringStiffness=0  SpringStiffnessUnits=N*m/deg  DampingCoefficient=0  DampingCoefficientUnits=N*m/(rad/s)  TorqueActuationMode=NoTorque  MotionActuationMode=ComputedMotion  SensePosition=off  SenseVelocity=off  SenseAcceleration=off  SenseTorqueForce=off  PositionTargetSpecify=off  PositionTargetPriority=High  PositionTargetValue=q(5,1)  PositionTargetValueUnits=rad  VelocityTargetSpecify=off  VelocityTargetPriority=High  VelocityTargetValue=100  VelocityTargetValueUnits=rad/s
  link_11 : Subsystem
  link_12 : Subsystem
  link_21 : Subsystem
  link_22 : Subsystem
  motor_inertia1 : sm_lib/Body Elements/Solid  InertiaType=Custom  Mass=0  MassUnits=kg  CenterOfMass=[0 0 0]  CenterOfMassUnits=m  MomentsOfInertia="[0  0 4.8e-5]"  MomentsOfInertiaUnits=kg*m^2  ProductsOfInertia=[0 0 0]  ProductsOfInertiaUnits=kg*m^2  BasedOnType=Density  Density=1000  DensityUnits=kg/m^3  DoExposeReferenceFrame=on  SerializedFrames=<Frames/>  GraphicType=FromGeometry  MarkerShape=Sphere  MarkerSize=10  GraphicVisPropType=SimpleVisualProperties  GraphicDiffuseColor=[1.0 1.0 0.0]  GraphicSpecularColor=[0.5 0.5 0.5 1.0]  GraphicAmbientColor=[0.15 0.15 0.15 1.0]  GraphicEmissiveColor=[0.0 0.0 0.0 1.0]  GraphicShininess=75  GraphicOpacity=1.0  GeometryShape=Sphere  RectangleSize=[1 1]  RectangleSizeUnits=m  BrickDimensions=[1 1 1]  BrickDimensionUnits=m  CylinderRadius=1  CylinderRadiusUnits=m  CylinderLength=1  CylinderLengthUnits=m  SphereRadius=1  SphereRadiusUnits=mm  EllipsoidRadii=[1 1 1]  EllipsoidRadiiUnits=m  ExtrusionCrossSection=[1 1; -1 1; -1 -1; 1 -1]  ExtrusionCrossSectionUnits=m  ExtrusionLength=1  ExtrusionLengthUnits=m  PolygonNumSides=3  PolygonOuterRadius=1  PolygonOuterRadiusUnits=m  ExtGeomFileType=STL  ExtGeomFileName=D:\PartsMechanism\propiedades\nema23_75mm_8mm.stl  ExtGeomFileUnits=mm  RevolutionCrossSection=[1 1; 1 -1; 2 -1; 2 1]  RevolutionCrossSectionUnits=m  RevolutionExtent=Full  RevolutionAngle=180  RevolutionAngleUnits=deg
  motor_inertia2 : sm_lib/Body Elements/Solid  InertiaType=Custom  Mass=0  MassUnits=kg  CenterOfMass=[0 0 0]  CenterOfMassUnits=m  MomentsOfInertia=[0 0 4.8e-5]  MomentsOfInertiaUnits=kg*m^2  ProductsOfInertia=[0 0 0]  ProductsOfInertiaUnits=kg*m^2  BasedOnType=Density  Density=1000  DensityUnits=kg/m^3  DoExposeReferenceFrame=on  SerializedFrames=<Frames/>  GraphicType=FromGeometry  MarkerShape=Sphere  MarkerSize=10  GraphicVisPropType=SimpleVisualProperties  GraphicDiffuseColor=[1.0 1.0 0.0]  GraphicSpecularColor=[0.5 0.5 0.5 1.0]  GraphicAmbientColor=[0.15 0.15 0.15 1.0]  GraphicEmissiveColor=[0.0 0.0 0.0 1.0]  GraphicShininess=75  GraphicOpacity=1.0  GeometryShape=Sphere  RectangleSize=[1 1]  RectangleSizeUnits=m  BrickDimensions=[1 1 1]  BrickDimensionUnits=m  CylinderRadius=1  CylinderRadiusUnits=m  CylinderLength=1  CylinderLengthUnits=m  SphereRadius=1  SphereRadiusUnits=mm  EllipsoidRadii=[1 1 1]  EllipsoidRadiiUnits=m  ExtrusionCrossSection=[1 1; -1 1; -1 -1; 1 -1]  ExtrusionCrossSectionUnits=m  ExtrusionLength=1  ExtrusionLengthUnits=m  PolygonNumSides=3  PolygonOuterRadius=1  PolygonOuterRadiusUnits=m  ExtGeomFileType=STL  ExtGeomFileName=D:\PartsMechanism\propiedades\nema23_75mm_8mm.stl  ExtGeomFileUnits=mm  RevolutionCrossSection=[1 1; 1 -1; 2 -1; 2 1]  RevolutionCrossSectionUnits=m  RevolutionExtent=Full  RevolutionAngle=180  RevolutionAngleUnits=deg
  world_2_base1 : sm_lib/Frames and Transforms/Rigid Transform  TranslationMethod=Cartesian  TranslationStandardOffset=0  TranslationLengthUnit=mm  TranslationStandardAxis=+Z  TranslationCartesianOffset=[-125 0 0]  TranslationROffset=0  TranslationROffsetUnits=m  TranslationZOffset=0  TranslationZOffsetUnits=m  TranslationThetaOffset=0  TranslationThetaOffsetUnits=deg  RotationMethod=None  RotationAngleUnits=deg  RotationStandardAxis=+Z  RotationAngle=0.0  RotationArbitraryAxis=[0 0 1]  FollAlignAxisA=+X  BaseAlignAxisA=+Y  FollAlignAxisB=+Y  BaseAlignAxisB=+Z  RotationSequenceAxes=FollowerAxes  RotationSequence=XYX  RotationSequenceAngles=[0 0 0]  RotationSequenceAnglesUnits=deg  RotationMatrix=[1 0 0; 0 1 0; 0 0 1]
  world_2_base2 : sm_lib/Frames and Transforms/Rigid Transform  TranslationMethod=Cartesian  TranslationStandardOffset=0  TranslationLengthUnit=mm  TranslationStandardAxis=+Z  TranslationCartesianOffset=[125 0 0]  TranslationROffset=0  TranslationROffsetUnits=m  TranslationZOffset=0  TranslationZOffsetUnits=m  TranslationThetaOffset=0  TranslationThetaOffsetUnits=deg  RotationMethod=None  RotationAngleUnits=deg  RotationStandardAxis=+Z  RotationAngle=0.0  RotationArbitraryAxis=[0 0 1]  FollAlignAxisA=+X  BaseAlignAxisA=+Y  FollAlignAxisB=+Y  BaseAlignAxisB=+Z  RotationSequenceAxes=FollowerAxes  RotationSequence=XYX  RotationSequenceAngles=[0 0 0]  RotationSequenceAnglesUnits=deg  RotationMatrix=[1 0 0; 0 1 0; 0 0 1]
  qa_o : Outport
  qda_o : Outport  Port=2
  qdda_o : Outport  Port=3
  wires:
  PS-Simulink Converter/1 -> Mux/1
  PS-Simulink Converter3/1 -> Mux1/2
  PS-Simulink Converter1/1 -> Mux/2
  PS-Simulink Converter2/1 -> Mux1/1
  Mux/1 -> qa_o/1
  Mux1/1 -> qda_o/1
  Ta/1 -> Demux3/1
  Demux3/1 -> Simulink-PS Converter2/1
  Demux3/2 -> Simulink-PS Converter3/1
  PS-Simulink Converter4/1 -> Mux2/1
  Mux2/1 -> qdda_o/1
  PS-Simulink Converter5/1 -> Mux2/2
  connections:
  joint12/LConn1 -- link_11/RConn1
  joint22/LConn1 -- link_21/RConn1
  World Frame/RConn1 -- world_2_base2/LConn1 -- Mechanism Configuration/RConn1 -- world_2_base1/LConn1 -- Solver Configuration/RConn1
  link_21/LConn1 -- joint21/RConn1 -- motor_inertia2/RConn1
  base1/RConn1 -- base1_2_joint11/LConn1 -- world_2_base1/RConn1
  base2_2_joint21/LConn1 -- base2/RConn1 -- world_2_base2/RConn1
  joint11/LConn1 -- base1_2_joint11/RConn1
  link_11/LConn1 -- motor_inertia1/RConn1 -- joint11/RConn1
  joint21/LConn1 -- base2_2_joint21/RConn1
  joint13/LConn1 -- end-effector/RConn1 -- link_12/RConn1
  link_22/RConn1 -- joint13/RConn1
  link_22/LConn1 -- joint22/RConn1
  link_12/LConn1 -- joint12/RConn1
  joint11/RConn2 -- PS-Simulink Converter/LConn1
  joint21/RConn2 -- PS-Simulink Converter1/LConn1
  joint21/RConn3 -- PS-Simulink Converter3/LConn1
  joint11/RConn3 -- PS-Simulink Converter2/LConn1
  Simulink-PS Converter2/RConn1 -- joint11/LConn2
  Simulink-PS Converter3/RConn1 -- joint21/LConn2
  PS-Simulink Converter5/LConn1 -- joint21/RConn4
  PS-Simulink Converter4/LConn1 -- joint11/RConn4

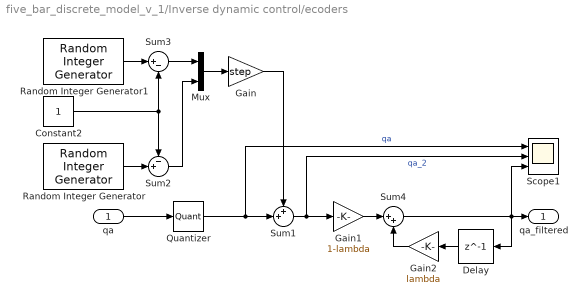
== system five_bar_discrete_model_v_1/Inverse dynamic control/ecoders ==
  qa : Inport
  Constant2 : Constant
  Delay : Delay  DelayLength=1  InitialCondition=[q0(1);q0(4)]
  Gain : Gain  Gain=step
  Gain1 : Gain  Gain=1-lambda
  Gain2 : Gain  Gain=lambda
  Mux : Mux  Inputs=2
  Quantizer : Quantizer  QuantizationInterval=step
  Random Integer Generator : commrandsrc3/Random Integer Generator  SetSize=3  SeedSource=Auto  Seed=0  SampleTime=0.1  SamplesPerFrame=1  OutputDataType=double  SimulateUsing=Interpreted execution
      settings: SourceProductName=Communications Toolbox
  Random Integer Generator1 : commrandsrc3/Random Integer Generator  SetSize=3  SeedSource=Auto  Seed=0  SampleTime=0.1  SamplesPerFrame=1  OutputDataType=double  SimulateUsing=Interpreted execution
      settings: SourceProductName=Communications Toolbox
  Scope1 : Scope  NumInputPorts=3
  Sum1 : Sum  Inputs=++|
  Sum2 : Sum  Inputs=-+|
  Sum3 : Sum  Inputs=|+-
  Sum4 : Sum  Inputs=|++
  qa_filtered : Outport
  wires:
  Mux/1 -> Gain/1
  Random Integer Generator/1 -> Sum2/2
  Sum3/1 -> Mux/1
  Sum1/1 -> Scope1/2, Gain1/1  "qa_2"
  Quantizer/1 -> Scope1/1, Sum1/2  "qa"
  Sum2/1 -> Mux/2
  Constant2/1 -> Sum3/2, Sum2/1
  Random Integer Generator1/1 -> Sum3/1
  Gain/1 -> Sum1/1
  Gain2/1 -> Sum4/2
  Gain1/1 -> Sum4/1
  Delay/1 -> Gain2/1
  Sum4/1 -> qa_filtered/1, Scope1/3, Delay/1
  qa/1 -> Quantizer/1

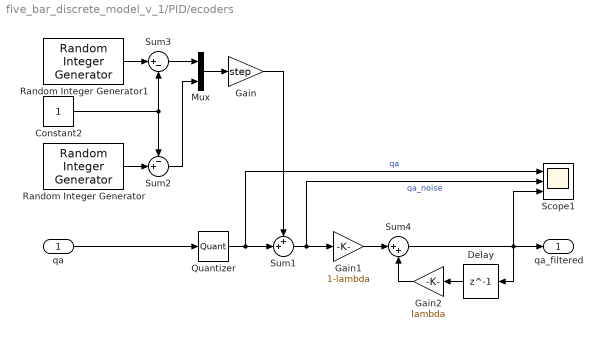
== system five_bar_discrete_model_v_1/PID/ecoders ==
  qa : Inport
  Constant2 : Constant
  Delay : Delay  DelayLength=1  InitialCondition=[q0(1);q0(4)]
  Gain : Gain  Gain=step
  Gain1 : Gain  Gain=1-lambda
  Gain2 : Gain  Gain=lambda
  Mux : Mux  Inputs=2
  Quantizer : Quantizer  QuantizationInterval=step
  Random Integer Generator : commrandsrc3/Random Integer Generator  SetSize=3  SeedSource=Auto  Seed=0  SampleTime=0.1  SamplesPerFrame=1  OutputDataType=double  SimulateUsing=Interpreted execution
      settings: SourceProductName=Communications Toolbox
  Random Integer Generator1 : commrandsrc3/Random Integer Generator  SetSize=3  SeedSource=Auto  Seed=0  SampleTime=0.1  SamplesPerFrame=1  OutputDataType=double  SimulateUsing=Interpreted execution
      settings: SourceProductName=Communications Toolbox
  Scope1 : Scope  NumInputPorts=3
  Sum1 : Sum  Inputs=++|
  Sum2 : Sum  Inputs=-+|
  Sum3 : Sum  Inputs=|+-
  Sum4 : Sum  Inputs=|++
  qa_filtered : Outport
  wires:
  Mux/1 -> Gain/1
  Random Integer Generator/1 -> Sum2/2
  Sum3/1 -> Mux/1
  Sum1/1 -> Gain1/1, Scope1/2  "qa_noise"
  Quantizer/1 -> Scope1/1, Sum1/2  "qa"
  Sum2/1 -> Mux/2
  Constant2/1 -> Sum3/2, Sum2/1
  Random Integer Generator1/1 -> Sum3/1
  Gain/1 -> Sum1/1
  Gain2/1 -> Sum4/2
  Gain1/1 -> Sum4/1
  Delay/1 -> Gain2/1
  Sum4/1 -> Delay/1, Scope1/3, qa_filtered/1
  qa/1 -> Quantizer/1

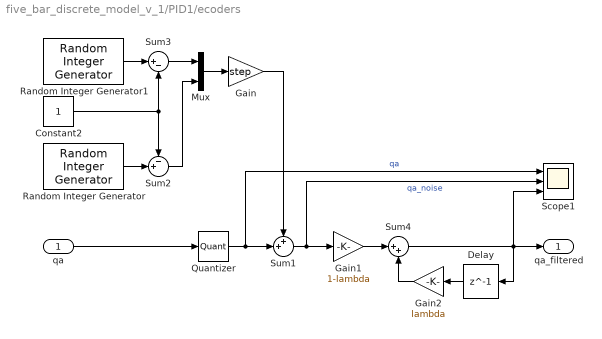
== system five_bar_discrete_model_v_1/PID1/ecoders ==
  qa : Inport
  Constant2 : Constant
  Delay : Delay  DelayLength=1  InitialCondition=[q0(1);q0(4)]
  Gain : Gain  Gain=step
  Gain1 : Gain  Gain=1-lambda
  Gain2 : Gain  Gain=lambda
  Mux : Mux  Inputs=2
  Quantizer : Quantizer  QuantizationInterval=step
  Random Integer Generator : commrandsrc3/Random Integer Generator  SetSize=3  SeedSource=Auto  Seed=0  SampleTime=0.1  SamplesPerFrame=1  OutputDataType=double  SimulateUsing=Interpreted execution
      settings: SourceProductName=Communications Toolbox
  Random Integer Generator1 : commrandsrc3/Random Integer Generator  SetSize=3  SeedSource=Auto  Seed=0  SampleTime=0.1  SamplesPerFrame=1  OutputDataType=double  SimulateUsing=Interpreted execution
      settings: SourceProductName=Communications Toolbox
  Scope1 : Scope  NumInputPorts=3
  Sum1 : Sum  Inputs=++|
  Sum2 : Sum  Inputs=-+|
  Sum3 : Sum  Inputs=|+-
  Sum4 : Sum  Inputs=|++
  qa_filtered : Outport
  wires:
  Mux/1 -> Gain/1
  Random Integer Generator/1 -> Sum2/2
  Sum3/1 -> Mux/1
  Sum1/1 -> Gain1/1, Scope1/2  "qa_noise"
  Quantizer/1 -> Scope1/1, Sum1/2  "qa"
  Sum2/1 -> Mux/2
  Constant2/1 -> Sum3/2, Sum2/1
  Random Integer Generator1/1 -> Sum3/1
  Gain/1 -> Sum1/1
  Gain2/1 -> Sum4/2
  Gain1/1 -> Sum4/1
  Delay/1 -> Gain2/1
  Sum4/1 -> Delay/1, Scope1/3, qa_filtered/1
  qa/1 -> Quantizer/1

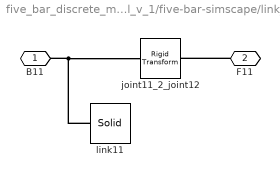
== system five_bar_discrete_model_v_1/five-bar-simscape/link_11 ==
  joint11_2_joint12 : sm_lib/Frames and Transforms/Rigid Transform  TranslationMethod=Cartesian  TranslationStandardOffset=0  TranslationLengthUnit=mm  TranslationStandardAxis=+Z  TranslationCartesianOffset=[205 -3 20]  TranslationROffset=0  TranslationROffsetUnits=m  TranslationZOffset=0  TranslationZOffsetUnits=m  TranslationThetaOffset=0  TranslationThetaOffsetUnits=deg  RotationMethod=None  RotationAngleUnits=deg  RotationStandardAxis=+Z  RotationAngle=0.0  RotationArbitraryAxis=[0 0 1]  FollAlignAxisA=+X  BaseAlignAxisA=+Y  FollAlignAxisB=+Y  BaseAlignAxisB=+Z  RotationSequenceAxes=FollowerAxes  RotationSequence=XYX  RotationSequenceAngles=[0 0 0]  RotationSequenceAnglesUnits=deg  RotationMatrix=[1 0 0; 0 1 0; 0 0 1]
  link11 : sm_lib/Body Elements/Solid  InertiaType=Custom  Mass=126  MassUnits=g  CenterOfMass=[0 10.25 0]  CenterOfMassUnits=cm  MomentsOfInertia="[17685.76 136.448  17738.24]"  MomentsOfInertiaUnits=g*cm^2  ProductsOfInertia=[0 0 0]  ProductsOfInertiaUnits=g*cm^2  BasedOnType=Density  Density=1000  DensityUnits=kg/m^3  DoExposeReferenceFrame=off  SerializedFrames=<Frames><Frame><Id>Frame1</Id><Value><Name>F1</Name><Origin><Source>ReferenceFrame</Source><FeatureName></FeatureName></Origin><PrimaryAxis><DefinedDirection>+Z</DefinedDirection><Source>ReferenceFrame</Source><SourceDirection>+Z</SourceDirection><FeatureName></FeatureName></PrimaryAxis><SecondaryAxis><DefinedDirection>+X</DefinedDirection><Source>ReferenceFrame</Source><SourceDirection>+Y</SourceDirection><FeatureName></FeatureName></SecondaryAxis></Value></Frame></Frames>  GraphicType=FromGeometry  MarkerShape=Sphere  MarkerSize=10  GraphicVisPropType=SimpleVisualProperties  GraphicDiffuseColor=[0.0 0.0 0.8]  GraphicSpecularColor=[0.5 0.5 0.5 1.0]  GraphicAmbientColor=[0.15 0.15 0.15 1.0]  GraphicEmissiveColor=[0.0 0.0 0.0 1.0]  GraphicShininess=75  GraphicOpacity=1.0  GeometryShape=FromFile  RectangleSize=[1 1]  RectangleSizeUnits=m  BrickDimensions=[1 1 1]  BrickDimensionUnits=m  CylinderRadius=1  CylinderRadiusUnits=m  CylinderLength=1  CylinderLengthUnits=m  SphereRadius=1  SphereRadiusUnits=m  EllipsoidRadii=[1 1 1]  EllipsoidRadiiUnits=m  ExtrusionCrossSection=[1 1; -1 1; -1 -1; 1 -1]  ExtrusionCrossSectionUnits=m  ExtrusionLength=1  ExtrusionLengthUnits=m  PolygonNumSides=3  PolygonOuterRadius=1  PolygonOuterRadiusUnits=m  ExtGeomFileType=STL  ExtGeomFileName=/home/jere/Documentos/simulacionPF/5-bar-model/meshes/link_11.stl  ExtGeomFileUnits=mm  RevolutionCrossSection=[1 1; 1 -1; 2 -1; 2 1]  RevolutionCrossSectionUnits=m  RevolutionExtent=Full  RevolutionAngle=180  RevolutionAngleUnits=deg
  B11 : PMIOPort  Side=Left
  F11 : PMIOPort  Port=2  Side=Right
  connections:
  F11/RConn1 -- joint11_2_joint12/RConn1
  link11/LConn1 -- B11/RConn1 -- joint11_2_joint12/LConn1

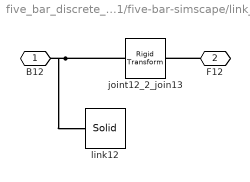
== system five_bar_discrete_model_v_1/five-bar-simscape/link_12 ==
  joint12_2_join13 : sm_lib/Frames and Transforms/Rigid Transform  TranslationMethod=Cartesian  TranslationStandardOffset=0  TranslationLengthUnit=mm  TranslationStandardAxis=+Z  TranslationCartesianOffset=[205 0 15]  TranslationROffset=0  TranslationROffsetUnits=m  TranslationZOffset=0  TranslationZOffsetUnits=m  TranslationThetaOffset=0  TranslationThetaOffsetUnits=deg  RotationMethod=None  RotationAngleUnits=deg  RotationStandardAxis=+Z  RotationAngle=0.0  RotationArbitraryAxis=[0 0 1]  FollAlignAxisA=+X  BaseAlignAxisA=+Y  FollAlignAxisB=+Y  BaseAlignAxisB=+Z  RotationSequenceAxes=FollowerAxes  RotationSequence=XYX  RotationSequenceAngles=[0 0 0]  RotationSequenceAnglesUnits=deg  RotationMatrix=[1 0 0; 0 1 0; 0 0 1]
  link12 : sm_lib/Body Elements/Solid  InertiaType=Custom  Mass=126  MassUnits=g  CenterOfMass=[0 10.25 0]  CenterOfMassUnits=cm  MomentsOfInertia="[17685.76 136.448  17738.24]"  MomentsOfInertiaUnits=g*cm^2  ProductsOfInertia=[0 0 0]  ProductsOfInertiaUnits=g*cm^2  BasedOnType=Density  Density=1000  DensityUnits=kg/m^3  DoExposeReferenceFrame=off  SerializedFrames=<Frames><Frame><Id>Frame1</Id><Value><Name>F1</Name><Origin><Source>ReferenceFrame</Source><FeatureName></FeatureName></Origin><PrimaryAxis><DefinedDirection>+Z</DefinedDirection><Source>ReferenceFrame</Source><SourceDirection>+Z</SourceDirection><FeatureName></FeatureName></PrimaryAxis><SecondaryAxis><DefinedDirection>+X</DefinedDirection><Source>ReferenceFrame</Source><SourceDirection>+Y</SourceDirection><FeatureName></FeatureName></SecondaryAxis></Value></Frame></Frames>  GraphicType=FromGeometry  MarkerShape=Sphere  MarkerSize=10  GraphicVisPropType=SimpleVisualProperties  GraphicDiffuseColor=[0.0 0.8 0.0]  GraphicSpecularColor=[0.5 0.5 0.5 1.0]  GraphicAmbientColor=[0.15 0.15 0.15 1.0]  GraphicEmissiveColor=[0.0 0.0 0.0 1.0]  GraphicShininess=75  GraphicOpacity=1.0  GeometryShape=FromFile  RectangleSize=[1 1]  RectangleSizeUnits=m  BrickDimensions=[1 1 1]  BrickDimensionUnits=m  CylinderRadius=1  CylinderRadiusUnits=m  CylinderLength=1  CylinderLengthUnits=m  SphereRadius=1  SphereRadiusUnits=m  EllipsoidRadii=[1 1 1]  EllipsoidRadiiUnits=m  ExtrusionCrossSection=[1 1; -1 1; -1 -1; 1 -1]  ExtrusionCrossSectionUnits=m  ExtrusionLength=1  ExtrusionLengthUnits=m  PolygonNumSides=3  PolygonOuterRadius=1  PolygonOuterRadiusUnits=m  ExtGeomFileType=STL  ExtGeomFileName=/home/jere/Documentos/simulacionPF/5-bar-model/meshes/link_12.stl  ExtGeomFileUnits=mm  RevolutionCrossSection=[1 1; 1 -1; 2 -1; 2 1]  RevolutionCrossSectionUnits=m  RevolutionExtent=Full  RevolutionAngle=180  RevolutionAngleUnits=deg
  B12 : PMIOPort  Side=Left
  F12 : PMIOPort  Port=2  Side=Right
  connections:
  F12/RConn1 -- joint12_2_join13/RConn1
  B12/RConn1 -- link12/LConn1 -- joint12_2_join13/LConn1
